simulink model "block_model"  (R2015b)
settings: Solver=ode45  StartTime=0.0  StopTime=10.0  RelTol=1e-3
values from neighbouring files (symbols this model uses):
  c = ureal('c',0.04,'Percentage',50)    [structured_uncertaines.m]
  k = ureal('k',4,'Percentage',50)    [structured_uncertaines.m]
  m = 1    [structured_uncertaines.m]
libraries: RCTblocks x2
settings Model: Creator=michele  LastModifiedBy=michele
settings DataIOCC: SaveFormat=Array
settings HardwareCC: ProdBitPerPointer=32  ProdLargestAtomicFloat=None  ProdIntDivRoundTo=Undefined  ProdEndianess=Unspecified  ProdWordSize=32  ProdHWDeviceType=32-bit Generic
settings GRTTargetCC: GeneratePreprocessorConditionals=Disable all
settings ConfigComp: CovModelRefEnable=Off  CovSFcnEnable=off

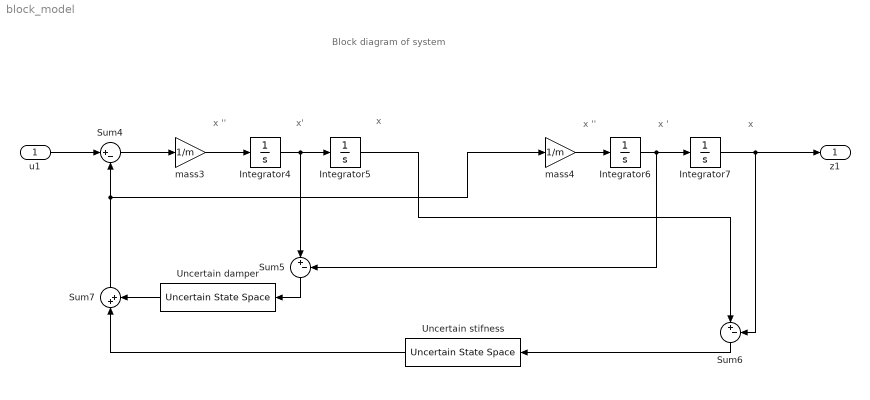
== system block_model ==
  note: Block diagram of system
  note: x
  note: x'
  note: x ''
  note: x ''
  note: x '
  note: x
  u1 : Inport
  Integrator{4..7} (4 alike) : Integrator
  Sum4 : Sum  Inputs=|+-
  Sum5 : Sum  Inputs=|+-
  Sum6 : Sum  Inputs=|+-
  Sum7 : Sum  Inputs=|++
  Uncertain damper : RCTblocks/Uncertain State Space  Tag=USS  USystem=ss(c)  UValue=[]  X0=[]  uX0=[]
  Uncertain stifness : RCTblocks/Uncertain State Space  Tag=USS  USystem=ss(k)  UValue=[]  X0=[]  uX0=[]
  mass3 : Gain  Gain=1/m
  mass4 : Gain  Gain=1/m
  z1 : Outport
  wires:
  Integrator4/1 -> Sum5/1, Integrator5/1
  Integrator6/1 -> Sum5/2, Integrator7/1
  Sum5/1 -> Uncertain damper/1
  Integrator5/1 -> Sum6/1
  Integrator7/1 -> z1/1, Sum6/2
  Sum6/1 -> Uncertain stifness/1
  Uncertain stifness/1 -> Sum7/1
  Sum7/1 -> Sum4/2, mass4/1
  mass3/1 -> Integrator4/1
  Sum4/1 -> mass3/1
  mass4/1 -> Integrator6/1
  u1/1 -> Sum4/1
  Uncertain damper/1 -> Sum7/2
